simulink model "PLANET_v2"  (R2018b)
settings: Solver=FixedStepAuto  StartTime=0.0  StopTime=span-1  FixedStep=0.1  RelTol=1e-3
undefined symbols (not defined in the file): CHP_eta_el, CHP_eta_th, CHP_Pn, control, dh_demand, DH_elB_Cap, DH_elB_eff, DH_gas_B_Cap, DH_gas_B_eff, DH_HP_Cap, DH_HP_COP, DiscIntNeverNeededParam, dt, h_elD, lhd_demand, LHD_elB_Cap, LHD_elB_eff, LHD_gas_B_Cap, LHD_gas_B_eff, LHD_HP_Cap, LHD_HP_COP, Liion_cap, Liion_charge, Liion_dis, Liion_eff_ch, Liion_eff_dis, PCI, PtG_cap, PtG_eta_elcto, PtG_eta_meth, PtG_eta_th, PVPower, RES_curtailment_on_off, tt, WindPower
libraries: simulink x1
(part 2 of 5)

== system PLANET_v2/Control /Li-ion control/Max discharge rate MW ==
  Discharge capacity : Constant  Value=Max_discharge
  Max battery discharge : Outport
  wires:
  Discharge capacity/1 -> Max battery discharge/1

== system PLANET_v2/Control /Production to Demand/If Action Subsystem ==
  Power produced : Inport
  Power demand : Inport  Port=2
  Action Port : ActionPort  ActionType=then
  Constant : Constant  Value=0
  Sum : Sum  Inputs=|+-
  New demand : Outport
  Surplus : Outport  Port=2
  wires:
  Power produced/1 -> Sum/1
  Sum/1 -> Surplus/1
  Power demand/1 -> Sum/2
  Constant/1 -> New demand/1

== system PLANET_v2/Control /Production to Demand/If Action Subsystem1 ==
  Power produced : Inport
  Power demand : Inport  Port=2
  Action Port : ActionPort  ActionType=else
  Constant : Constant  Value=0
  Sum : Sum  Inputs=-+|
  Surplus : Outport
  New demand : Outport  Port=2
  wires:
  Sum/1 -> New demand/1
  Constant/1 -> Surplus/1
  Power demand/1 -> Sum/2
  Power produced/1 -> Sum/1

== system PLANET_v2/Control /Production to Demand1/If Action Subsystem ==
  Power produced : Inport
  Power demand : Inport  Port=2
  Action Port : ActionPort  ActionType=then
  Constant : Constant  Value=0
  Sum : Sum  Inputs=|+-
  New demand : Outport
  Surplus : Outport  Port=2
  wires:
  Power produced/1 -> Sum/1
  Sum/1 -> Surplus/1
  Power demand/1 -> Sum/2
  Constant/1 -> New demand/1

== system PLANET_v2/Control /Production to Demand1/If Action Subsystem1 ==
  Power produced : Inport
  Power demand : Inport  Port=2
  Action Port : ActionPort  ActionType=else
  Constant : Constant  Value=0
  Sum : Sum  Inputs=-+|
  Surplus : Outport
  New demand : Outport  Port=2
  wires:
  Sum/1 -> New demand/1
  Constant/1 -> Surplus/1
  Power demand/1 -> Sum/2
  Power produced/1 -> Sum/1

== system PLANET_v2/Control /Production to Demand2/If Action Subsystem ==
  Power produced : Inport
  Power demand : Inport  Port=2
  Action Port : ActionPort  ActionType=then
  Constant : Constant  Value=0
  Sum : Sum  Inputs=|+-
  New demand : Outport
  Surplus : Outport  Port=2
  wires:
  Power produced/1 -> Sum/1
  Sum/1 -> Surplus/1
  Power demand/1 -> Sum/2
  Constant/1 -> New demand/1

== system PLANET_v2/Control /Production to Demand2/If Action Subsystem1 ==
  Power produced : Inport
  Power demand : Inport  Port=2
  Action Port : ActionPort  ActionType=else
  Constant : Constant  Value=0
  Sum : Sum  Inputs=-+|
  Surplus : Outport
  New demand : Outport  Port=2
  wires:
  Sum/1 -> New demand/1
  Constant/1 -> Surplus/1
  Power demand/1 -> Sum/2
  Power produced/1 -> Sum/1

== system PLANET_v2/Control /Surplus dispacth/0: Li-ion P2G P2H1 ==
  Surplus MW : Inport
  " Li-ion charge MWh" : Inport  Port=2
  Th demand MW : Inport  Port=3
  Action Port : ActionPort  ActionType=then
  Li-ion control2 : Subsystem  mask{eff_charge=Liion_eff_ch, eff_discharge=Liion_eff_dis, SoC_MAX=100, SoC_MIN=0, Capacity=Liion_cap, Initial_SoC=50, Max_charge=Liion_charge, Max_discharge=Liion_dis}
      mask prompts: eff_charge "charging efficiency [%]"; eff_discharge "discharging efficiency [%]"; SoC_MAX "Maximum state of charge [%]"; SoC_MIN "Minimum state of charge [%]"; Capacity "Capacity [MWh]"; Initial_SoC "Initial State of charge [%]"; Max_charge "Max charge [MW]"; Max_discharge "Max discharge [MW]"
  P2G control : Subsystem  mask{PtG_capacity=PtG_cap, eff_electrolyser=PtG_eta_elcto, eff_methanizer=PtG_eta_meth, eff_thermal=PtG_eta_th, PCI=PCI}
      mask prompts: PtG_capacity "PtG capacity"; eff_electrolyser "Electrolyser efficiency"; eff_methanizer "Methanizer efficiency"; eff_thermal "Thermal efficiency"; PCI "PCI Mehtane MWh/kg"
  P2H : Subsystem  mask{HP_LHD_cap=LHD_HP_Cap, HP_LHD_COP=LHD_HP_COP, elB_LHD_cap=LHD_elB_Cap, elB_LHD_eff=LHD_elB_eff, HP_DH_cap=DH_HP_Cap, HP_DH_COP=DH_HP_COP, elB_DH_cap=DH_elB_Cap, elB_DH_eff=DH_elB_eff}
      mask prompts: HP_LHD_cap "LHD HP Capacity"; HP_LHD_COP "LHD HP COP"; elB_LHD_cap "LHD el boiler Capacity"; elB_LHD_eff "LHD el boiler efficiency"; HP_DH_cap "DH HP Capacity"; HP_DH_COP "DH HP COP"; elB_DH_cap "DH el boiler Capacity"; elB_DH_eff "DH el boiler efficiency"
  New surplus MW : Outport
  New th dem MW : Outport  Port=2
  Li-ion el input MW : Outport  Port=3
  P2G el input MW : Outport  Port=4
  P2H el input MW : Outport  Port=5
  wires:
  P2G control/1(New surplus MW) -> P2H/2(Surplus MW)
  Li-ion control2/1(New surplus MW) -> P2G control/1(Surplus MW)
  P2G control/2(P2G el input MW) -> P2G el input MW/1
  Li-ion control2/2(Battery el input MW) -> Li-ion el input MW/1
  " Li-ion charge MWh"/1 -> Li-ion control2/2(Initial charge MWh)
  P2H/3(New th dem) -> New th dem MW/1
  P2H/1(P2H el input) -> P2H el input MW/1
  P2H/2(New surplus MW) -> New surplus MW/1
  Th demand MW/1 -> P2H/1(Th demand)
  Surplus MW/1 -> Li-ion control2/1(Surplus MW)

== system PLANET_v2/Control /Surplus dispacth/1: Li-ion P2H P2G ==
  Surplus MW : Inport
  " Li-ion charge MWh" : Inport  Port=2
  Th demand MW : Inport  Port=3
  Action Port : ActionPort  ActionType=elseif
  Li-ion control2 : Subsystem  mask{eff_charge=Liion_eff_ch, eff_discharge=Liion_eff_dis, SoC_MAX=100, SoC_MIN=0, Capacity=Liion_cap, Initial_SoC=50, Max_charge=Liion_charge, Max_discharge=Liion_dis}
      mask prompts: eff_charge "charging efficiency [%]"; eff_discharge "discharging efficiency [%]"; SoC_MAX "Maximum state of charge [%]"; SoC_MIN "Minimum state of charge [%]"; Capacity "Capacity [MWh]"; Initial_SoC "Initial State of charge [%]"; Max_charge "Max charge [MW]"; Max_discharge "Max discharge [MW]"
  P2G control : Subsystem  mask{PtG_capacity=PtG_cap, eff_electrolyser=PtG_eta_elcto, eff_methanizer=PtG_eta_meth, eff_thermal=PtG_eta_th, PCI=PCI}
      mask prompts: PtG_capacity "PtG capacity"; eff_electrolyser "Electrolyser efficiency"; eff_methanizer "Methanizer efficiency"; eff_thermal "Thermal efficiency"; PCI "PCI Mehtane MWh/kg"
  P2H : Subsystem  mask{HP_LHD_cap=LHD_HP_Cap, HP_LHD_COP=LHD_HP_COP, elB_LHD_cap=LHD_elB_Cap, elB_LHD_eff=LHD_elB_eff, HP_DH_cap=DH_HP_Cap, HP_DH_COP=DH_HP_COP, elB_DH_cap=DH_elB_Cap, elB_DH_eff=DH_elB_eff}
      mask prompts: HP_LHD_cap "LHD HP Capacity"; HP_LHD_COP "LHD HP COP"; elB_LHD_cap "LHD el boiler Capacity"; elB_LHD_eff "LHD el boiler efficiency"; HP_DH_cap "DH HP Capacity"; HP_DH_COP "DH HP COP"; elB_DH_cap "DH el boiler Capacity"; elB_DH_eff "DH el boiler efficiency"
  New surplus MW : Outport
  New th dem MW : Outport  Port=2
  Li-ion el input MW : Outport  Port=3
  P2G el input MW : Outport  Port=4
  P2H el input MW : Outport  Port=5
  wires:
  P2G control/1(New surplus MW) -> New surplus MW/1
  P2H/2(New surplus MW) -> P2G control/1(Surplus MW)
  Li-ion control2/1(New surplus MW) -> P2H/2(Surplus MW)
  Surplus MW/1 -> Li-ion control2/1(Surplus MW)
  Th demand MW/1 -> P2H/1(Th demand)
  P2H/1(P2H el input) -> P2H el input MW/1
  P2H/3(New th dem) -> New th dem MW/1
  " Li-ion charge MWh"/1 -> Li-ion control2/2(Initial charge MWh)
  Li-ion control2/2(Battery el input MW) -> Li-ion el input MW/1
  P2G control/2(P2G el input MW) -> P2G el input MW/1

== system PLANET_v2/Control /Surplus dispacth/2: P2G Li-ion P2H ==
  Surplus MW : Inport
  " Li-ion charge MWh" : Inport  Port=2
  Th demand MW : Inport  Port=3
  Action Port : ActionPort  ActionType=elseif
  Li-ion control2 : Subsystem  mask{eff_charge=Liion_eff_ch, eff_discharge=Liion_eff_dis, SoC_MAX=100, SoC_MIN=0, Capacity=Liion_cap, Initial_SoC=50, Max_charge=Liion_charge, Max_discharge=Liion_dis}
      mask prompts: eff_charge "charging efficiency [%]"; eff_discharge "discharging efficiency [%]"; SoC_MAX "Maximum state of charge [%]"; SoC_MIN "Minimum state of charge [%]"; Capacity "Capacity [MWh]"; Initial_SoC "Initial State of charge [%]"; Max_charge "Max charge [MW]"; Max_discharge "Max discharge [MW]"
  P2G control : Subsystem  mask{PtG_capacity=PtG_cap, eff_electrolyser=PtG_eta_elcto, eff_methanizer=PtG_eta_meth, eff_thermal=PtG_eta_th, PCI=PCI}
      mask prompts: PtG_capacity "PtG capacity"; eff_electrolyser "Electrolyser efficiency"; eff_methanizer "Methanizer efficiency"; eff_thermal "Thermal efficiency"; PCI "PCI Mehtane MWh/kg"
  P2H : Subsystem  mask{HP_LHD_cap=LHD_HP_Cap, HP_LHD_COP=LHD_HP_COP, elB_LHD_cap=LHD_elB_Cap, elB_LHD_eff=LHD_elB_eff, HP_DH_cap=DH_HP_Cap, HP_DH_COP=DH_HP_COP, elB_DH_cap=DH_elB_Cap, elB_DH_eff=DH_elB_eff}
      mask prompts: HP_LHD_cap "LHD HP Capacity"; HP_LHD_COP "LHD HP COP"; elB_LHD_cap "LHD el boiler Capacity"; elB_LHD_eff "LHD el boiler efficiency"; HP_DH_cap "DH HP Capacity"; HP_DH_COP "DH HP COP"; elB_DH_cap "DH el boiler Capacity"; elB_DH_eff "DH el boiler efficiency"
  New surplus MW : Outport
  New th dem MW : Outport  Port=2
  Li-ion el input MW : Outport  Port=3
  P2G el input MW : Outport  Port=4
  P2H el input MW : Outport  Port=5
  wires:
  Li-ion control2/1(New surplus MW) -> P2H/2(Surplus MW)
  P2G control/1(New surplus MW) -> Li-ion control2/1(Surplus MW)
  Surplus MW/1 -> P2G control/1(Surplus MW)
  Th demand MW/1 -> P2H/1(Th demand)
  P2H/2(New surplus MW) -> New surplus MW/1
  P2H/1(P2H el input) -> P2H el input MW/1
  P2H/3(New th dem) -> New th dem MW/1
  " Li-ion charge MWh"/1 -> Li-ion control2/2(Initial charge MWh)
  Li-ion control2/2(Battery el input MW) -> Li-ion el input MW/1
  P2G control/2(P2G el input MW) -> P2G el input MW/1

== system PLANET_v2/Control /Surplus dispacth/3: P2G P2H Li-ion ==
  Surplus MW : Inport
  " Li-ion charge MWh" : Inport  Port=2
  Th demand MW : Inport  Port=3
  Action Port : ActionPort  ActionType=elseif
  Li-ion control2 : Subsystem  mask{eff_charge=Liion_eff_ch, eff_discharge=Liion_eff_dis, SoC_MAX=100, SoC_MIN=0, Capacity=Liion_cap, Initial_SoC=50, Max_charge=Liion_charge, Max_discharge=Liion_dis}
      mask prompts: eff_charge "charging efficiency [%]"; eff_discharge "discharging efficiency [%]"; SoC_MAX "Maximum state of charge [%]"; SoC_MIN "Minimum state of charge [%]"; Capacity "Capacity [MWh]"; Initial_SoC "Initial State of charge [%]"; Max_charge "Max charge [MW]"; Max_discharge "Max discharge [MW]"
  P2G control : Subsystem  mask{PtG_capacity=PtG_cap, eff_electrolyser=PtG_eta_elcto, eff_methanizer=PtG_eta_meth, eff_thermal=PtG_eta_th, PCI=PCI}
      mask prompts: PtG_capacity "PtG capacity"; eff_electrolyser "Electrolyser efficiency"; eff_methanizer "Methanizer efficiency"; eff_thermal "Thermal efficiency"; PCI "PCI Mehtane MWh/kg"
  P2H : Subsystem  mask{HP_LHD_cap=LHD_HP_Cap, HP_LHD_COP=LHD_HP_COP, elB_LHD_cap=LHD_elB_Cap, elB_LHD_eff=LHD_elB_eff, HP_DH_cap=DH_HP_Cap, HP_DH_COP=DH_HP_COP, elB_DH_cap=DH_elB_Cap, elB_DH_eff=DH_elB_eff}
      mask prompts: HP_LHD_cap "LHD HP Capacity"; HP_LHD_COP "LHD HP COP"; elB_LHD_cap "LHD el boiler Capacity"; elB_LHD_eff "LHD el boiler efficiency"; HP_DH_cap "DH HP Capacity"; HP_DH_COP "DH HP COP"; elB_DH_cap "DH el boiler Capacity"; elB_DH_eff "DH el boiler efficiency"
  New surplus MW : Outport
  New th dem MW : Outport  Port=2
  Li-ion el input MW : Outport  Port=3
  P2G el input MW : Outport  Port=4
  P2H el input MW : Outport  Port=5
  wires:
  Li-ion control2/1(New surplus MW) -> New surplus MW/1
  P2H/2(New surplus MW) -> Li-ion control2/1(Surplus MW)
  P2G control/1(New surplus MW) -> P2H/2(Surplus MW)
  Surplus MW/1 -> P2G control/1(Surplus MW)
  Th demand MW/1 -> P2H/1(Th demand)
  P2H/1(P2H el input) -> P2H el input MW/1
  P2H/3(New th dem) -> New th dem MW/1
  " Li-ion charge MWh"/1 -> Li-ion control2/2(Initial charge MWh)
  Li-ion control2/2(Battery el input MW) -> Li-ion el input MW/1
  P2G control/2(P2G el input MW) -> P2G el input MW/1

== system PLANET_v2/Control /Surplus dispacth/4: P2H Li-ion P2G ==
  Surplus MW : Inport
  " Li-ion charge MWh" : Inport  Port=2
  Th demand MW : Inport  Port=3
  Action Port : ActionPort  ActionType=elseif
  Li-ion control2 : Subsystem  mask{eff_charge=Liion_eff_ch, eff_discharge=Liion_eff_dis, SoC_MAX=100, SoC_MIN=0, Capacity=Liion_cap, Initial_SoC=50, Max_charge=Liion_charge, Max_discharge=Liion_dis}
      mask prompts: eff_charge "charging efficiency [%]"; eff_discharge "discharging efficiency [%]"; SoC_MAX "Maximum state of charge [%]"; SoC_MIN "Minimum state of charge [%]"; Capacity "Capacity [MWh]"; Initial_SoC "Initial State of charge [%]"; Max_charge "Max charge [MW]"; Max_discharge "Max discharge [MW]"
  P2G control : Subsystem  mask{PtG_capacity=PtG_cap, eff_electrolyser=PtG_eta_elcto, eff_methanizer=PtG_eta_meth, eff_thermal=PtG_eta_th, PCI=PCI}
      mask prompts: PtG_capacity "PtG capacity"; eff_electrolyser "Electrolyser efficiency"; eff_methanizer "Methanizer efficiency"; eff_thermal "Thermal efficiency"; PCI "PCI Mehtane MWh/kg"
  P2H : Subsystem  mask{HP_LHD_cap=LHD_HP_Cap, HP_LHD_COP=LHD_HP_COP, elB_LHD_cap=LHD_elB_Cap, elB_LHD_eff=LHD_elB_eff, HP_DH_cap=DH_HP_Cap, HP_DH_COP=DH_HP_COP, elB_DH_cap=DH_elB_Cap, elB_DH_eff=DH_elB_eff}
      mask prompts: HP_LHD_cap "LHD HP Capacity"; HP_LHD_COP "LHD HP COP"; elB_LHD_cap "LHD el boiler Capacity"; elB_LHD_eff "LHD el boiler efficiency"; HP_DH_cap "DH HP Capacity"; HP_DH_COP "DH HP COP"; elB_DH_cap "DH el boiler Capacity"; elB_DH_eff "DH el boiler efficiency"
  New surplus MW : Outport
  New th dem MW : Outport  Port=2
  Li-ion el input MW : Outport  Port=3
  P2G el input MW : Outport  Port=4
  P2H el input MW : Outport  Port=5
  wires:
  Surplus MW/1 -> P2H/2(Surplus MW)
  P2G control/1(New surplus MW) -> New surplus MW/1
  Li-ion control2/1(New surplus MW) -> P2G control/1(Surplus MW)
  P2H/2(New surplus MW) -> Li-ion control2/1(Surplus MW)
  Th demand MW/1 -> P2H/1(Th demand)
  P2H/1(P2H el input) -> P2H el input MW/1
  P2H/3(New th dem) -> New th dem MW/1
  " Li-ion charge MWh"/1 -> Li-ion control2/2(Initial charge MWh)
  Li-ion control2/2(Battery el input MW) -> Li-ion el input MW/1
  P2G control/2(P2G el input MW) -> P2G el input MW/1

== system PLANET_v2/Control /Surplus dispacth/5: P2H P2G Li-ion  ==
  Surplus MW : Inport
  " Li-ion charge MWh" : Inport  Port=2
  Th demand MW : Inport  Port=3
  Action Port : ActionPort  ActionType=elseif
  Li-ion control2 : Subsystem  mask{eff_charge=Liion_eff_ch, eff_discharge=Liion_eff_dis, SoC_MAX=100, SoC_MIN=0, Capacity=Liion_cap, Initial_SoC=50, Max_charge=Liion_charge, Max_discharge=Liion_dis}
      mask prompts: eff_charge "charging efficiency [%]"; eff_discharge "discharging efficiency [%]"; SoC_MAX "Maximum state of charge [%]"; SoC_MIN "Minimum state of charge [%]"; Capacity "Capacity [MWh]"; Initial_SoC "Initial State of charge [%]"; Max_charge "Max charge [MW]"; Max_discharge "Max discharge [MW]"
  P2G control : Subsystem  mask{PtG_capacity=PtG_cap, eff_electrolyser=PtG_eta_elcto, eff_methanizer=PtG_eta_meth, eff_thermal=PtG_eta_th, PCI=PCI}
      mask prompts: PtG_capacity "PtG capacity"; eff_electrolyser "Electrolyser efficiency"; eff_methanizer "Methanizer efficiency"; eff_thermal "Thermal efficiency"; PCI "PCI Mehtane MWh/kg"
  P2H : Subsystem  mask{HP_LHD_cap=LHD_HP_Cap, HP_LHD_COP=LHD_HP_COP, elB_LHD_cap=LHD_elB_Cap, elB_LHD_eff=LHD_elB_eff, HP_DH_cap=DH_HP_Cap, HP_DH_COP=DH_HP_COP, elB_DH_cap=DH_elB_Cap, elB_DH_eff=DH_elB_eff}
      mask prompts: HP_LHD_cap "LHD HP Capacity"; HP_LHD_COP "LHD HP COP"; elB_LHD_cap "LHD el boiler Capacity"; elB_LHD_eff "LHD el boiler efficiency"; HP_DH_cap "DH HP Capacity"; HP_DH_COP "DH HP COP"; elB_DH_cap "DH el boiler Capacity"; elB_DH_eff "DH el boiler efficiency"
  New surplus MW : Outport
  New th dem MW : Outport  Port=2
  Li-ion el input MW : Outport  Port=3
  P2G el input MW : Outport  Port=4
  P2H el input MW : Outport  Port=5
  wires:
  P2H/3(New th dem) -> New th dem MW/1
  Li-ion control2/1(New surplus MW) -> New surplus MW/1
  Surplus MW/1 -> P2H/2(Surplus MW)
  P2H/2(New surplus MW) -> P2G control/1(Surplus MW)
  P2G control/1(New surplus MW) -> Li-ion control2/1(Surplus MW)
  Th demand MW/1 -> P2H/1(Th demand)
  P2H/1(P2H el input) -> P2H el input MW/1
  " Li-ion charge MWh"/1 -> Li-ion control2/2(Initial charge MWh)
  Li-ion control2/2(Battery el input MW) -> Li-ion el input MW/1
  P2G control/2(P2G el input MW) -> P2G el input MW/1

== system PLANET_v2/Gas boiler (DH)/DH Gas Boiler block/Boiler ==
  Fuel mass : Inport
  Divide1 : Product  Inputs=***
  Efficiency : Constant  Value=eff/100
  PCI MWh/kg2 : Constant  Value=PCI
  Thermal power : Outport
  wires:
  Divide1/1 -> Thermal power/1
  Efficiency/1 -> Divide1/3
  Fuel mass/1 -> Divide1/1
  PCI MWh/kg2/1 -> Divide1/2

== system PLANET_v2/Gas boiler (LH)/LH Gas Boiler block/Boiler ==
  Fuel mass : Inport
  Divide1 : Product  Inputs=***
  Efficiency : Constant  Value=eff/100
  PCI MWh/kg2 : Constant  Value=PCI
  Thermal power : Outport
  wires:
  Divide1/1 -> Thermal power/1
  Efficiency/1 -> Divide1/3
  Fuel mass/1 -> Divide1/1
  PCI MWh/kg2/1 -> Divide1/2

== system PLANET_v2/Liion/Li-ion /State of charge calulation ==
  Charge : Inport
  Capacity : Constant  Value=Capacity
  Constant1 : Constant
  Divide : Product  Inputs=*/
  Gain : Gain  Gain=100
  Switch : Switch  Criteria=u2 > Threshold
  State of Charege : Outport
  wires:
  Charge/1 -> Divide/1
  Gain/1 -> State of Charege/1
  Divide/1 -> Gain/1
  Switch/1 -> Divide/2
  Capacity/1 -> Switch/2, Switch/1
  Constant1/1 -> Switch/3

== system PLANET_v2/Liion/Li-ion /Subsystem ==
  El input : Inport
  El output : Inport  Port=2
  Accumulation : DiscreteIntegrator  InitialConditionSource=external  ICPrevOutput=DiscIntNeverNeededParam  ICPrevScaledInput=DiscIntNeverNeededParam
  Initial Charge t0 : Subsystem
  Power to Energy : Subsystem
  Sum : Sum  Inputs=|++
  Sum1 : Sum  Inputs=+-|
  "Initial charge " : Outport
  New charge : Outport  Port=2
  wires:
  Sum/1 -> New charge/1
  Accumulation/1 -> "Initial charge "/1, Sum/2  "Charge inside the battery before the new input"
  Initial Charge t0/1(IC) -> Accumulation/2
  El input/1 -> Sum1/1
  El output/1 -> Sum1/2
  Power to Energy/1(Energy) -> Sum/1, Accumulation/1
  Sum1/1 -> Power to Energy/1(Power)

== system PLANET_v2/P2G/P2G/Max P2G electric input ==
  P2G capacity : Constant  Value=PtG_capacity
  Max P2G input : Outport
  wires:
  P2G capacity/1 -> Max P2G input/1

== system PLANET_v2/Subsystem/Environment/Analogic control1 ==
  Value : Inport
  Constant : Constant  Value=125.39682539683
  Constant1 : Constant  Value=0
  Gain : Gain  Gain=1/100
  Product : Product
  Switch : Switch  Criteria=u2 > Threshold
  Modifed value : Outport
  wires:
  Gain/1 -> Product/1
  Value/1 -> Switch/3, Product/2
  Switch/1 -> Modifed value/1
  Product/1 -> Switch/1
  Constant1/1 -> Switch/2
  Constant/1 -> Gain/1

== system PLANET_v2/Subsystem/Environment/Analogic control2 ==
  Value : Inport
  Constant : Constant  Value=100
  Constant1 : Constant  Value=0
  Gain : Gain  Gain=1/100
  Product : Product
  Switch : Switch  Criteria=u2 > Threshold
  Modifed value : Outport
  wires:
  Gain/1 -> Product/1
  Value/1 -> Switch/3, Product/2
  Switch/1 -> Modifed value/1
  Product/1 -> Switch/1
  Constant1/1 -> Switch/2
  Constant/1 -> Gain/1

== system PLANET_v2/Subsystem/Environment/Analogic control3 ==
  Value : Inport
  Constant : Constant  Value=100
  Constant1 : Constant  Value=0
  Gain : Gain  Gain=1/100
  Product : Product
  Switch : Switch  Criteria=u2 > Threshold
  Modifed value : Outport
  wires:
  Gain/1 -> Product/1
  Value/1 -> Switch/3, Product/2
  Switch/1 -> Modifed value/1
  Product/1 -> Switch/1
  Constant1/1 -> Switch/2
  Constant/1 -> Gain/1

== system PLANET_v2/Control /Surplus dispacth/0: Li-ion P2G P2H1/Li-ion control2 ==
  Surplus MW : Inport
  Initial charge MWh : Inport  Port=2
  " " : If  NumInputs=3  IfExpression=u1 == 0  ElseIfExpressions=(u1 <= u2) & (u1<=u3), u2<=u3
  Bypassed surp : Merge  Inputs=4
  Ch eff : Gain  Gain=100/eff_charge
  Charge to battery : Merge  Inputs=4
  Energy to Power : Subsystem
  Free Battery MWh : Subsystem
  If Action Subsystem : Subsystem  TreatAsAtomicUnit=on
  If Action Subsystem1 : Subsystem  TreatAsAtomicUnit=on
  If Action Subsystem2 : Subsystem  TreatAsAtomicUnit=on
  If Action Subsystem4 : Subsystem  TreatAsAtomicUnit=on
  MAX charge MW : Subsystem
  New surplus MW : Outport
  Battery el input MW : Outport  Port=2
  wires:
  Ch eff/1 -> " "/3, If Action Subsystem4/1(free battery)
  Energy to Power/1(Power) -> Ch eff/1
  Initial charge MWh/1 -> Free Battery MWh/1(In1)
  If Action Subsystem1/1(Bypassed surplus) -> Bypassed surp/2
  " "/2 -> If Action Subsystem1/Action
  If Action Subsystem/2(To battery) -> Charge to battery/1
  Free Battery MWh/1(Free space) -> Energy to Power/1(Energy)
  If Action Subsystem2/2(To battery) -> Charge to battery/3
  Surplus MW/1 -> If Action Subsystem1/1(Surplus), " "/1, If Action Subsystem2/2(Surplus), If Action Subsystem4/2(Surplus)
  " "/1 -> If Action Subsystem/Action
  If Action Subsystem4/2(To battery) -> Charge to battery/4
  " "/3 -> If Action Subsystem2/Action
  If Action Subsystem2/1(Bypassed surplus) -> Bypassed surp/3
  " "/4 -> If Action Subsystem4/Action
  Bypassed surp/1 -> New surplus MW/1  "Not accumulated energy surplus"
  If Action Subsystem1/2(To battery) -> Charge to battery/2
  Charge to battery/1 -> Battery el input MW/1  "Surplus energy send to the battery"
  MAX charge MW/1(Max battery charge) -> " "/2, If Action Subsystem2/1(Max charge)
  If Action Subsystem/1(Bypassed surplus) -> Bypassed surp/1
  If Action Subsystem4/1(Bypassed surplus) -> Bypassed surp/4

== system PLANET_v2/Control /Surplus dispacth/0: Li-ion P2G P2H1/P2G control ==
  Surplus MW : Inport
  If : If  NumInputs=2  IfExpression=u1 <= 0  ElseIfExpressions=u1 <= u2
  If Action Subsystem : Subsystem  TreatAsAtomicUnit=on
  If Action Subsystem1 : Subsystem  TreatAsAtomicUnit=on
  If Action Subsystem2 : Subsystem  TreatAsAtomicUnit=on
  Max P2G electric input : Subsystem
  Merge1 : Merge  Inputs=3
  Sum : Sum  Inputs=|+-
  New surplus MW : Outport
  P2G el input MW : Outport  Port=2
  wires:
  Max P2G electric input/1(Max PtG input) -> If/2
  If/1 -> If Action Subsystem2/Action
  If/3 -> If Action Subsystem/Action
  If Action Subsystem1/1(New surplus) -> Merge1/2
  Surplus MW/1 -> Sum/1, If Action Subsystem/1(Surplus), If/1
  If Action Subsystem/1(New surplus) -> Merge1/3
  If Action Subsystem2/1(New surplus) -> Merge1/1
  Merge1/1 -> Sum/2, New surplus MW/1
  If/2 -> If Action Subsystem1/Action
  Sum/1 -> P2G el input MW/1

== system PLANET_v2/Control /Surplus dispacth/0: Li-ion P2G P2H1/P2H ==
  Th demand : Inport
  Surplus MW : Inport  Port=2
  Bus Creator : BusCreator  Inputs=4
  Bus Creator1 : BusCreator  Inputs=2
  Bus Selector : BusSelector  OutputSignals=Lh dem,Dh dem
  Electric boiler DH : Subsystem  mask{th_eff=elB_DH_eff, Cap=elB_DH_cap}
      mask prompts: Cap "Capacity MW"
  Electric boiler LHD : Subsystem  mask{th_eff=elB_LHD_eff, Cap=elB_LHD_cap}
      mask prompts: Cap "Capacity MW"
  HEAT PUMP DH : Subsystem  mask{COP=HP_DH_COP, Cap=HP_DH_cap}
      mask prompts: Cap "Capacity MW"
  HEAT PUMP local : Subsystem  mask{COP=HP_LHD_COP, Cap=HP_LHD_cap}
      mask prompts: Cap "Capacity MW"
  P2H el input : Outport
  New surplus MW : Outport  Port=2
  New th dem : Outport  Port=3
  wires:
  Surplus MW/1 -> HEAT PUMP local/1(Surplus)
  Bus Selector/2 -> HEAT PUMP DH/2(th demand)  "<Dh dem>"
  HEAT PUMP local/2(New surplus) -> HEAT PUMP DH/1(Surplus)
  HEAT PUMP DH/2(New surplus) -> Electric boiler LHD/1(Surplus)
  HEAT PUMP local/3(New th_d) -> Electric boiler LHD/2(th demand)
  Electric boiler LHD/2(New surplus) -> Electric boiler DH/1(Surplus)
  HEAT PUMP DH/3(New th_d) -> Electric boiler DH/2(th demand)
  Electric boiler DH/2(New surplus) -> New surplus MW/1
  Electric boiler LHD/3(New th_d) -> Bus Creator1/1  "Lh dem"
  Electric boiler DH/3(New th_d) -> Bus Creator1/2  "Dh dem"
  HEAT PUMP local/1(el cons) -> Bus Creator/1  "HP (LH) el input"
  HEAT PUMP DH/1(el cons) -> Bus Creator/2  "HP (DH) el input"
  Electric boiler LHD/1(el cons) -> Bus Creator/3  "elB (LH) el input"
  Electric boiler DH/1(el cons) -> Bus Creator/4  "elB (DH) el input"
  Bus Creator/1 -> P2H el input/1
  Th demand/1 -> Bus Selector/1
  Bus Selector/1 -> HEAT PUMP local/2(th demand)  "<Lh dem>"
  Bus Creator1/1 -> New th dem/1  "Th dem"

== system PLANET_v2/Control /Surplus dispacth/1: Li-ion P2H P2G/Li-ion control2 ==
  Surplus MW : Inport
  Initial charge MWh : Inport  Port=2
  " " : If  NumInputs=3  IfExpression=u1 == 0  ElseIfExpressions=(u1 <= u2) & (u1<=u3), u2<=u3
  Bypassed surp : Merge  Inputs=4
  Ch eff : Gain  Gain=100/eff_charge
  Charge to battery : Merge  Inputs=4
  Energy to Power : Subsystem
  Free Battery MWh : Subsystem
  If Action Subsystem : Subsystem  TreatAsAtomicUnit=on
  If Action Subsystem1 : Subsystem  TreatAsAtomicUnit=on
  If Action Subsystem2 : Subsystem  TreatAsAtomicUnit=on
  If Action Subsystem4 : Subsystem  TreatAsAtomicUnit=on
  MAX charge MW : Subsystem
  New surplus MW : Outport
  Battery el input MW : Outport  Port=2
  wires:
  Ch eff/1 -> " "/3, If Action Subsystem4/1(free battery)
  Energy to Power/1(Power) -> Ch eff/1
  Initial charge MWh/1 -> Free Battery MWh/1(In1)
  If Action Subsystem1/1(Bypassed surplus) -> Bypassed surp/2
  " "/2 -> If Action Subsystem1/Action
  If Action Subsystem/2(To battery) -> Charge to battery/1
  Free Battery MWh/1(Free space) -> Energy to Power/1(Energy)
  If Action Subsystem2/2(To battery) -> Charge to battery/3
  Surplus MW/1 -> If Action Subsystem1/1(Surplus), " "/1, If Action Subsystem2/2(Surplus), If Action Subsystem4/2(Surplus)
  " "/1 -> If Action Subsystem/Action
  If Action Subsystem4/2(To battery) -> Charge to battery/4
  " "/3 -> If Action Subsystem2/Action
  If Action Subsystem2/1(Bypassed surplus) -> Bypassed surp/3
  " "/4 -> If Action Subsystem4/Action
  Bypassed surp/1 -> New surplus MW/1  "Not accumulated energy surplus"
  If Action Subsystem1/2(To battery) -> Charge to battery/2
  Charge to battery/1 -> Battery el input MW/1  "Surplus energy send to the battery"
  MAX charge MW/1(Max battery charge) -> " "/2, If Action Subsystem2/1(Max charge)
  If Action Subsystem/1(Bypassed surplus) -> Bypassed surp/1
  If Action Subsystem4/1(Bypassed surplus) -> Bypassed surp/4

== system PLANET_v2/Control /Surplus dispacth/1: Li-ion P2H P2G/P2G control ==
  Surplus MW : Inport
  If : If  NumInputs=2  IfExpression=u1 <= 0  ElseIfExpressions=u1 <= u2
  If Action Subsystem : Subsystem  TreatAsAtomicUnit=on
  If Action Subsystem1 : Subsystem  TreatAsAtomicUnit=on
  If Action Subsystem2 : Subsystem  TreatAsAtomicUnit=on
  Max P2G electric input : Subsystem
  Merge1 : Merge  Inputs=3
  Sum : Sum  Inputs=|+-
  New surplus MW : Outport
  P2G el input MW : Outport  Port=2
  wires:
  Max P2G electric input/1(Max PtG input) -> If/2
  If/1 -> If Action Subsystem2/Action
  If/3 -> If Action Subsystem/Action
  If Action Subsystem1/1(New surplus) -> Merge1/2
  Surplus MW/1 -> Sum/1, If Action Subsystem/1(Surplus), If/1
  If Action Subsystem/1(New surplus) -> Merge1/3
  If Action Subsystem2/1(New surplus) -> Merge1/1
  Merge1/1 -> Sum/2, New surplus MW/1
  If/2 -> If Action Subsystem1/Action
  Sum/1 -> P2G el input MW/1

== system PLANET_v2/Control /Surplus dispacth/1: Li-ion P2H P2G/P2H ==
  Th demand : Inport
  Surplus MW : Inport  Port=2
  Bus Creator : BusCreator  Inputs=4
  Bus Creator1 : BusCreator  Inputs=2
  Bus Selector : BusSelector  OutputSignals=Lh dem,Dh dem
  Electric boiler DH : Subsystem  mask{th_eff=elB_DH_eff, Cap=elB_DH_cap}
      mask prompts: Cap "Capacity MW"
  Electric boiler LHD : Subsystem  mask{th_eff=elB_LHD_eff, Cap=elB_LHD_cap}
      mask prompts: Cap "Capacity MW"
  HEAT PUMP DH : Subsystem  mask{COP=HP_DH_COP, Cap=HP_DH_cap}
      mask prompts: Cap "Capacity MW"
  HEAT PUMP local : Subsystem  mask{COP=HP_LHD_COP, Cap=HP_LHD_cap}
      mask prompts: Cap "Capacity MW"
  P2H el input : Outport
  New surplus MW : Outport  Port=2
  New th dem : Outport  Port=3
  wires:
  Bus Creator1/1 -> New th dem/1  "Th dem"
  Bus Selector/1 -> HEAT PUMP local/2(th demand)  "<Lh dem>"
  Th demand/1 -> Bus Selector/1
  Bus Creator/1 -> P2H el input/1
  Electric boiler DH/1(el cons) -> Bus Creator/4  "elB (DH) el input"
  Electric boiler LHD/1(el cons) -> Bus Creator/3  "elB (LH) el input"
  HEAT PUMP DH/1(el cons) -> Bus Creator/2  "HP (DH) el input"
  HEAT PUMP local/1(el cons) -> Bus Creator/1  "HP (LH) el input"
  Electric boiler DH/3(New th_d) -> Bus Creator1/2  "Dh dem"
  Electric boiler LHD/3(New th_d) -> Bus Creator1/1  "Lh dem"
  Electric boiler DH/2(New surplus) -> New surplus MW/1
  HEAT PUMP DH/3(New th_d) -> Electric boiler DH/2(th demand)
  Electric boiler LHD/2(New surplus) -> Electric boiler DH/1(Surplus)
  HEAT PUMP local/3(New th_d) -> Electric boiler LHD/2(th demand)
  HEAT PUMP DH/2(New surplus) -> Electric boiler LHD/1(Surplus)
  HEAT PUMP local/2(New surplus) -> HEAT PUMP DH/1(Surplus)
  Bus Selector/2 -> HEAT PUMP DH/2(th demand)  "<Dh dem>"
  Surplus MW/1 -> HEAT PUMP local/1(Surplus)

== system PLANET_v2/Control /Surplus dispacth/2: P2G Li-ion P2H/Li-ion control2 ==
  Surplus MW : Inport
  Initial charge MWh : Inport  Port=2
  " " : If  NumInputs=3  IfExpression=u1 == 0  ElseIfExpressions=(u1 <= u2) & (u1<=u3), u2<=u3
  Bypassed surp : Merge  Inputs=4
  Ch eff : Gain  Gain=100/eff_charge
  Charge to battery : Merge  Inputs=4
  Energy to Power : Subsystem
  Free Battery MWh : Subsystem
  If Action Subsystem : Subsystem  TreatAsAtomicUnit=on
  If Action Subsystem1 : Subsystem  TreatAsAtomicUnit=on
  If Action Subsystem2 : Subsystem  TreatAsAtomicUnit=on
  If Action Subsystem4 : Subsystem  TreatAsAtomicUnit=on
  MAX charge MW : Subsystem
  New surplus MW : Outport
  Battery el input MW : Outport  Port=2
  wires:
  Ch eff/1 -> " "/3, If Action Subsystem4/1(free battery)
  Energy to Power/1(Power) -> Ch eff/1
  Initial charge MWh/1 -> Free Battery MWh/1(In1)
  If Action Subsystem1/1(Bypassed surplus) -> Bypassed surp/2
  " "/2 -> If Action Subsystem1/Action
  If Action Subsystem/2(To battery) -> Charge to battery/1
  Free Battery MWh/1(Free space) -> Energy to Power/1(Energy)
  If Action Subsystem2/2(To battery) -> Charge to battery/3
  Surplus MW/1 -> If Action Subsystem1/1(Surplus), " "/1, If Action Subsystem2/2(Surplus), If Action Subsystem4/2(Surplus)
  " "/1 -> If Action Subsystem/Action
  If Action Subsystem4/2(To battery) -> Charge to battery/4
  " "/3 -> If Action Subsystem2/Action
  If Action Subsystem2/1(Bypassed surplus) -> Bypassed surp/3
  " "/4 -> If Action Subsystem4/Action
  Bypassed surp/1 -> New surplus MW/1  "Not accumulated energy surplus"
  If Action Subsystem1/2(To battery) -> Charge to battery/2
  Charge to battery/1 -> Battery el input MW/1  "Surplus energy send to the battery"
  MAX charge MW/1(Max battery charge) -> " "/2, If Action Subsystem2/1(Max charge)
  If Action Subsystem/1(Bypassed surplus) -> Bypassed surp/1
  If Action Subsystem4/1(Bypassed surplus) -> Bypassed surp/4

== system PLANET_v2/Control /Surplus dispacth/2: P2G Li-ion P2H/P2G control ==
  Surplus MW : Inport
  If : If  NumInputs=2  IfExpression=u1 <= 0  ElseIfExpressions=u1 <= u2
  If Action Subsystem : Subsystem  TreatAsAtomicUnit=on
  If Action Subsystem1 : Subsystem  TreatAsAtomicUnit=on
  If Action Subsystem2 : Subsystem  TreatAsAtomicUnit=on
  Max P2G electric input : Subsystem
  Merge1 : Merge  Inputs=3
  Sum : Sum  Inputs=|+-
  New surplus MW : Outport
  P2G el input MW : Outport  Port=2
  wires:
  Max P2G electric input/1(Max PtG input) -> If/2
  If/1 -> If Action Subsystem2/Action
  If/3 -> If Action Subsystem/Action
  If Action Subsystem1/1(New surplus) -> Merge1/2
  Surplus MW/1 -> Sum/1, If Action Subsystem/1(Surplus), If/1
  If Action Subsystem/1(New surplus) -> Merge1/3
  If Action Subsystem2/1(New surplus) -> Merge1/1
  Merge1/1 -> Sum/2, New surplus MW/1
  If/2 -> If Action Subsystem1/Action
  Sum/1 -> P2G el input MW/1

== system PLANET_v2/Control /Surplus dispacth/2: P2G Li-ion P2H/P2H ==
  Th demand : Inport
  Surplus MW : Inport  Port=2
  Bus Creator : BusCreator  Inputs=4
  Bus Creator1 : BusCreator  Inputs=2
  Bus Selector : BusSelector  OutputSignals=Lh dem,Dh dem
  Electric boiler DH : Subsystem  mask{th_eff=elB_DH_eff, Cap=elB_DH_cap}
      mask prompts: Cap "Capacity MW"
  Electric boiler LHD : Subsystem  mask{th_eff=elB_LHD_eff, Cap=elB_LHD_cap}
      mask prompts: Cap "Capacity MW"
  HEAT PUMP DH : Subsystem  mask{COP=HP_DH_COP, Cap=HP_DH_cap}
      mask prompts: Cap "Capacity MW"
  HEAT PUMP local : Subsystem  mask{COP=HP_LHD_COP, Cap=HP_LHD_cap}
      mask prompts: Cap "Capacity MW"
  P2H el input : Outport
  New surplus MW : Outport  Port=2
  New th dem : Outport  Port=3
  wires:
  Bus Creator1/1 -> New th dem/1  "Th dem"
  Bus Selector/1 -> HEAT PUMP local/2(th demand)  "<Lh dem>"
  Th demand/1 -> Bus Selector/1
  Bus Creator/1 -> P2H el input/1
  Electric boiler DH/1(el cons) -> Bus Creator/4  "elB (DH) el input"
  Electric boiler LHD/1(el cons) -> Bus Creator/3  "elB (LH) el input"
  HEAT PUMP DH/1(el cons) -> Bus Creator/2  "HP (DH) el input"
  HEAT PUMP local/1(el cons) -> Bus Creator/1  "HP (LH) el input"
  Electric boiler DH/3(New th_d) -> Bus Creator1/2  "Dh dem"
  Electric boiler LHD/3(New th_d) -> Bus Creator1/1  "Lh dem"
  Electric boiler DH/2(New surplus) -> New surplus MW/1
  HEAT PUMP DH/3(New th_d) -> Electric boiler DH/2(th demand)
  Electric boiler LHD/2(New surplus) -> Electric boiler DH/1(Surplus)
  HEAT PUMP local/3(New th_d) -> Electric boiler LHD/2(th demand)
  HEAT PUMP DH/2(New surplus) -> Electric boiler LHD/1(Surplus)
  HEAT PUMP local/2(New surplus) -> HEAT PUMP DH/1(Surplus)
  Bus Selector/2 -> HEAT PUMP DH/2(th demand)  "<Dh dem>"
  Surplus MW/1 -> HEAT PUMP local/1(Surplus)

== system PLANET_v2/Control /Surplus dispacth/3: P2G P2H Li-ion/Li-ion control2 ==
  Surplus MW : Inport
  Initial charge MWh : Inport  Port=2
  " " : If  NumInputs=3  IfExpression=u1 == 0  ElseIfExpressions=(u1 <= u2) & (u1<=u3), u2<=u3
  Bypassed surp : Merge  Inputs=4
  Ch eff : Gain  Gain=100/eff_charge
  Charge to battery : Merge  Inputs=4
  Energy to Power : Subsystem
  Free Battery MWh : Subsystem
  If Action Subsystem : Subsystem  TreatAsAtomicUnit=on
  If Action Subsystem1 : Subsystem  TreatAsAtomicUnit=on
  If Action Subsystem2 : Subsystem  TreatAsAtomicUnit=on
  If Action Subsystem4 : Subsystem  TreatAsAtomicUnit=on
  MAX charge MW : Subsystem
  New surplus MW : Outport
  Battery el input MW : Outport  Port=2
  wires:
  Ch eff/1 -> " "/3, If Action Subsystem4/1(free battery)
  Energy to Power/1(Power) -> Ch eff/1
  Initial charge MWh/1 -> Free Battery MWh/1(In1)
  If Action Subsystem1/1(Bypassed surplus) -> Bypassed surp/2
  " "/2 -> If Action Subsystem1/Action
  If Action Subsystem/2(To battery) -> Charge to battery/1
  Free Battery MWh/1(Free space) -> Energy to Power/1(Energy)
  If Action Subsystem2/2(To battery) -> Charge to battery/3
  Surplus MW/1 -> If Action Subsystem1/1(Surplus), " "/1, If Action Subsystem2/2(Surplus), If Action Subsystem4/2(Surplus)
  " "/1 -> If Action Subsystem/Action
  If Action Subsystem4/2(To battery) -> Charge to battery/4
  " "/3 -> If Action Subsystem2/Action
  If Action Subsystem2/1(Bypassed surplus) -> Bypassed surp/3
  " "/4 -> If Action Subsystem4/Action
  Bypassed surp/1 -> New surplus MW/1  "Not accumulated energy surplus"
  If Action Subsystem1/2(To battery) -> Charge to battery/2
  Charge to battery/1 -> Battery el input MW/1  "Surplus energy send to the battery"
  MAX charge MW/1(Max battery charge) -> " "/2, If Action Subsystem2/1(Max charge)
  If Action Subsystem/1(Bypassed surplus) -> Bypassed surp/1
  If Action Subsystem4/1(Bypassed surplus) -> Bypassed surp/4

== system PLANET_v2/Control /Surplus dispacth/3: P2G P2H Li-ion/P2G control ==
  Surplus MW : Inport
  If : If  NumInputs=2  IfExpression=u1 <= 0  ElseIfExpressions=u1 <= u2
  If Action Subsystem : Subsystem  TreatAsAtomicUnit=on
  If Action Subsystem1 : Subsystem  TreatAsAtomicUnit=on
  If Action Subsystem2 : Subsystem  TreatAsAtomicUnit=on
  Max P2G electric input : Subsystem
  Merge1 : Merge  Inputs=3
  Sum : Sum  Inputs=|+-
  New surplus MW : Outport
  P2G el input MW : Outport  Port=2
  wires:
  Max P2G electric input/1(Max PtG input) -> If/2
  If/1 -> If Action Subsystem2/Action
  If/3 -> If Action Subsystem/Action
  If Action Subsystem1/1(New surplus) -> Merge1/2
  Surplus MW/1 -> Sum/1, If Action Subsystem/1(Surplus), If/1
  If Action Subsystem/1(New surplus) -> Merge1/3
  If Action Subsystem2/1(New surplus) -> Merge1/1
  Merge1/1 -> Sum/2, New surplus MW/1
  If/2 -> If Action Subsystem1/Action
  Sum/1 -> P2G el input MW/1

== system PLANET_v2/Control /Surplus dispacth/3: P2G P2H Li-ion/P2H ==
  Th demand : Inport
  Surplus MW : Inport  Port=2
  Bus Creator : BusCreator  Inputs=4
  Bus Creator1 : BusCreator  Inputs=2
  Bus Selector : BusSelector  OutputSignals=Lh dem,Dh dem
  Electric boiler DH : Subsystem  mask{th_eff=elB_DH_eff, Cap=elB_DH_cap}
      mask prompts: Cap "Capacity MW"
  Electric boiler LHD : Subsystem  mask{th_eff=elB_LHD_eff, Cap=elB_LHD_cap}
      mask prompts: Cap "Capacity MW"
  HEAT PUMP DH : Subsystem  mask{COP=HP_DH_COP, Cap=HP_DH_cap}
      mask prompts: Cap "Capacity MW"
  HEAT PUMP local : Subsystem  mask{COP=HP_LHD_COP, Cap=HP_LHD_cap}
      mask prompts: Cap "Capacity MW"
  P2H el input : Outport
  New surplus MW : Outport  Port=2
  New th dem : Outport  Port=3
  wires:
  Bus Creator1/1 -> New th dem/1  "Th dem"
  Bus Selector/1 -> HEAT PUMP local/2(th demand)  "<Lh dem>"
  Th demand/1 -> Bus Selector/1
  Bus Creator/1 -> P2H el input/1
  Electric boiler DH/1(el cons) -> Bus Creator/4  "elB (DH) el input"
  Electric boiler LHD/1(el cons) -> Bus Creator/3  "elB (LH) el input"
  HEAT PUMP DH/1(el cons) -> Bus Creator/2  "HP (DH) el input"
  HEAT PUMP local/1(el cons) -> Bus Creator/1  "HP (LH) el input"
  Electric boiler DH/3(New th_d) -> Bus Creator1/2  "Dh dem"
  Electric boiler LHD/3(New th_d) -> Bus Creator1/1  "Lh dem"
  Electric boiler DH/2(New surplus) -> New surplus MW/1
  HEAT PUMP DH/3(New th_d) -> Electric boiler DH/2(th demand)
  Electric boiler LHD/2(New surplus) -> Electric boiler DH/1(Surplus)
  HEAT PUMP local/3(New th_d) -> Electric boiler LHD/2(th demand)
  HEAT PUMP DH/2(New surplus) -> Electric boiler LHD/1(Surplus)
  HEAT PUMP local/2(New surplus) -> HEAT PUMP DH/1(Surplus)
  Bus Selector/2 -> HEAT PUMP DH/2(th demand)  "<Dh dem>"
  Surplus MW/1 -> HEAT PUMP local/1(Surplus)

== system PLANET_v2/Control /Surplus dispacth/4: P2H Li-ion P2G/Li-ion control2 ==
  Surplus MW : Inport
  Initial charge MWh : Inport  Port=2
  " " : If  NumInputs=3  IfExpression=u1 == 0  ElseIfExpressions=(u1 <= u2) & (u1<=u3), u2<=u3
  Bypassed surp : Merge  Inputs=4
  Ch eff : Gain  Gain=100/eff_charge
  Charge to battery : Merge  Inputs=4
  Energy to Power : Subsystem
  Free Battery MWh : Subsystem
  If Action Subsystem : Subsystem  TreatAsAtomicUnit=on
  If Action Subsystem1 : Subsystem  TreatAsAtomicUnit=on
  If Action Subsystem2 : Subsystem  TreatAsAtomicUnit=on
  If Action Subsystem4 : Subsystem  TreatAsAtomicUnit=on
  MAX charge MW : Subsystem
  New surplus MW : Outport
  Battery el input MW : Outport  Port=2
  wires:
  Ch eff/1 -> " "/3, If Action Subsystem4/1(free battery)
  Energy to Power/1(Power) -> Ch eff/1
  Initial charge MWh/1 -> Free Battery MWh/1(In1)
  If Action Subsystem1/1(Bypassed surplus) -> Bypassed surp/2
  " "/2 -> If Action Subsystem1/Action
  If Action Subsystem/2(To battery) -> Charge to battery/1
  Free Battery MWh/1(Free space) -> Energy to Power/1(Energy)
  If Action Subsystem2/2(To battery) -> Charge to battery/3
  Surplus MW/1 -> If Action Subsystem1/1(Surplus), " "/1, If Action Subsystem2/2(Surplus), If Action Subsystem4/2(Surplus)
  " "/1 -> If Action Subsystem/Action
  If Action Subsystem4/2(To battery) -> Charge to battery/4
  " "/3 -> If Action Subsystem2/Action
  If Action Subsystem2/1(Bypassed surplus) -> Bypassed surp/3
  " "/4 -> If Action Subsystem4/Action
  Bypassed surp/1 -> New surplus MW/1  "Not accumulated energy surplus"
  If Action Subsystem1/2(To battery) -> Charge to battery/2
  Charge to battery/1 -> Battery el input MW/1  "Surplus energy send to the battery"
  MAX charge MW/1(Max battery charge) -> " "/2, If Action Subsystem2/1(Max charge)
  If Action Subsystem/1(Bypassed surplus) -> Bypassed surp/1
  If Action Subsystem4/1(Bypassed surplus) -> Bypassed surp/4

== system PLANET_v2/Control /Surplus dispacth/4: P2H Li-ion P2G/P2G control ==
  Surplus MW : Inport
  If : If  NumInputs=2  IfExpression=u1 <= 0  ElseIfExpressions=u1 <= u2
  If Action Subsystem : Subsystem  TreatAsAtomicUnit=on
  If Action Subsystem1 : Subsystem  TreatAsAtomicUnit=on
  If Action Subsystem2 : Subsystem  TreatAsAtomicUnit=on
  Max P2G electric input : Subsystem
  Merge1 : Merge  Inputs=3
  Sum : Sum  Inputs=|+-
  New surplus MW : Outport
  P2G el input MW : Outport  Port=2
  wires:
  Max P2G electric input/1(Max PtG input) -> If/2
  If/1 -> If Action Subsystem2/Action
  If/3 -> If Action Subsystem/Action
  If Action Subsystem1/1(New surplus) -> Merge1/2
  Surplus MW/1 -> Sum/1, If Action Subsystem/1(Surplus), If/1
  If Action Subsystem/1(New surplus) -> Merge1/3
  If Action Subsystem2/1(New surplus) -> Merge1/1
  Merge1/1 -> Sum/2, New surplus MW/1
  If/2 -> If Action Subsystem1/Action
  Sum/1 -> P2G el input MW/1

== system PLANET_v2/Control /Surplus dispacth/4: P2H Li-ion P2G/P2H ==
  Th demand : Inport
  Surplus MW : Inport  Port=2
  Bus Creator : BusCreator  Inputs=4
  Bus Creator1 : BusCreator  Inputs=2
  Bus Selector : BusSelector  OutputSignals=Lh dem,Dh dem
  Electric boiler DH : Subsystem  mask{th_eff=elB_DH_eff, Cap=elB_DH_cap}
      mask prompts: Cap "Capacity MW"
  Electric boiler LHD : Subsystem  mask{th_eff=elB_LHD_eff, Cap=elB_LHD_cap}
      mask prompts: Cap "Capacity MW"
  HEAT PUMP DH : Subsystem  mask{COP=HP_DH_COP, Cap=HP_DH_cap}
      mask prompts: Cap "Capacity MW"
  HEAT PUMP local : Subsystem  mask{COP=HP_LHD_COP, Cap=HP_LHD_cap}
      mask prompts: Cap "Capacity MW"
  P2H el input : Outport
  New surplus MW : Outport  Port=2
  New th dem : Outport  Port=3
  wires:
  Bus Creator1/1 -> New th dem/1  "Th dem"
  Bus Selector/1 -> HEAT PUMP local/2(th demand)  "<Lh dem>"
  Th demand/1 -> Bus Selector/1
  Bus Creator/1 -> P2H el input/1
  Electric boiler DH/1(el cons) -> Bus Creator/4  "elB (DH) el input"
  Electric boiler LHD/1(el cons) -> Bus Creator/3  "elB (LH) el input"
  HEAT PUMP DH/1(el cons) -> Bus Creator/2  "HP (DH) el input"
  HEAT PUMP local/1(el cons) -> Bus Creator/1  "HP (LH) el input"
  Electric boiler DH/3(New th_d) -> Bus Creator1/2  "Dh dem"
  Electric boiler LHD/3(New th_d) -> Bus Creator1/1  "Lh dem"
  Electric boiler DH/2(New surplus) -> New surplus MW/1
  HEAT PUMP DH/3(New th_d) -> Electric boiler DH/2(th demand)
  Electric boiler LHD/2(New surplus) -> Electric boiler DH/1(Surplus)
  HEAT PUMP local/3(New th_d) -> Electric boiler LHD/2(th demand)
  HEAT PUMP DH/2(New surplus) -> Electric boiler LHD/1(Surplus)
  HEAT PUMP local/2(New surplus) -> HEAT PUMP DH/1(Surplus)
  Bus Selector/2 -> HEAT PUMP DH/2(th demand)  "<Dh dem>"
  Surplus MW/1 -> HEAT PUMP local/1(Surplus)

== system PLANET_v2/Control /Surplus dispacth/5: P2H P2G Li-ion /Li-ion control2 ==
  Surplus MW : Inport
  Initial charge MWh : Inport  Port=2
  " " : If  NumInputs=3  IfExpression=u1 == 0  ElseIfExpressions=(u1 <= u2) & (u1<=u3), u2<=u3
  Bypassed surp : Merge  Inputs=4
  Ch eff : Gain  Gain=100/eff_charge
  Charge to battery : Merge  Inputs=4
  Energy to Power : Subsystem
  Free Battery MWh : Subsystem
  If Action Subsystem : Subsystem  TreatAsAtomicUnit=on
  If Action Subsystem1 : Subsystem  TreatAsAtomicUnit=on
  If Action Subsystem2 : Subsystem  TreatAsAtomicUnit=on
  If Action Subsystem4 : Subsystem  TreatAsAtomicUnit=on
  MAX charge MW : Subsystem
  New surplus MW : Outport
  Battery el input MW : Outport  Port=2
  wires:
  Ch eff/1 -> " "/3, If Action Subsystem4/1(free battery)
  Energy to Power/1(Power) -> Ch eff/1
  Initial charge MWh/1 -> Free Battery MWh/1(In1)
  If Action Subsystem1/1(Bypassed surplus) -> Bypassed surp/2
  " "/2 -> If Action Subsystem1/Action
  If Action Subsystem/2(To battery) -> Charge to battery/1
  Free Battery MWh/1(Free space) -> Energy to Power/1(Energy)
  If Action Subsystem2/2(To battery) -> Charge to battery/3
  Surplus MW/1 -> If Action Subsystem1/1(Surplus), " "/1, If Action Subsystem2/2(Surplus), If Action Subsystem4/2(Surplus)
  " "/1 -> If Action Subsystem/Action
  If Action Subsystem4/2(To battery) -> Charge to battery/4
  " "/3 -> If Action Subsystem2/Action
  If Action Subsystem2/1(Bypassed surplus) -> Bypassed surp/3
  " "/4 -> If Action Subsystem4/Action
  Bypassed surp/1 -> New surplus MW/1  "Not accumulated energy surplus"
  If Action Subsystem1/2(To battery) -> Charge to battery/2
  Charge to battery/1 -> Battery el input MW/1  "Surplus energy send to the battery"
  MAX charge MW/1(Max battery charge) -> " "/2, If Action Subsystem2/1(Max charge)
  If Action Subsystem/1(Bypassed surplus) -> Bypassed surp/1
  If Action Subsystem4/1(Bypassed surplus) -> Bypassed surp/4

== system PLANET_v2/Control /Surplus dispacth/5: P2H P2G Li-ion /P2G control ==
  Surplus MW : Inport
  If : If  NumInputs=2  IfExpression=u1 <= 0  ElseIfExpressions=u1 <= u2
  If Action Subsystem : Subsystem  TreatAsAtomicUnit=on
  If Action Subsystem1 : Subsystem  TreatAsAtomicUnit=on
  If Action Subsystem2 : Subsystem  TreatAsAtomicUnit=on
  Max P2G electric input : Subsystem
  Merge1 : Merge  Inputs=3
  Sum : Sum  Inputs=|+-
  New surplus MW : Outport
  P2G el input MW : Outport  Port=2
  wires:
  Max P2G electric input/1(Max PtG input) -> If/2
  If/1 -> If Action Subsystem2/Action
  If/3 -> If Action Subsystem/Action
  If Action Subsystem1/1(New surplus) -> Merge1/2
  Surplus MW/1 -> Sum/1, If Action Subsystem/1(Surplus), If/1
  If Action Subsystem/1(New surplus) -> Merge1/3
  If Action Subsystem2/1(New surplus) -> Merge1/1
  Merge1/1 -> Sum/2, New surplus MW/1
  If/2 -> If Action Subsystem1/Action
  Sum/1 -> P2G el input MW/1

== system PLANET_v2/Control /Surplus dispacth/5: P2H P2G Li-ion /P2H ==
  Th demand : Inport
  Surplus MW : Inport  Port=2
  Bus Creator : BusCreator  Inputs=4
  Bus Creator1 : BusCreator  Inputs=2
  Bus Selector : BusSelector  OutputSignals=Lh dem,Dh dem
  Electric boiler DH : Subsystem  mask{th_eff=elB_DH_eff, Cap=elB_DH_cap}
      mask prompts: Cap "Capacity MW"
  Electric boiler LHD : Subsystem  mask{th_eff=elB_LHD_eff, Cap=elB_LHD_cap}
      mask prompts: Cap "Capacity MW"
  HEAT PUMP DH : Subsystem  mask{COP=HP_DH_COP, Cap=HP_DH_cap}
      mask prompts: Cap "Capacity MW"
  HEAT PUMP local : Subsystem  mask{COP=HP_LHD_COP, Cap=HP_LHD_cap}
      mask prompts: Cap "Capacity MW"
  P2H el input : Outport
  New surplus MW : Outport  Port=2
  New th dem : Outport  Port=3
  wires:
  Bus Creator1/1 -> New th dem/1  "Th dem"
  Bus Selector/1 -> HEAT PUMP local/2(th demand)  "<Lh dem>"
  Th demand/1 -> Bus Selector/1
  Bus Creator/1 -> P2H el input/1
  Electric boiler DH/1(el cons) -> Bus Creator/4  "elB (DH) el input"
  Electric boiler LHD/1(el cons) -> Bus Creator/3  "elB (LH) el input"
  HEAT PUMP DH/1(el cons) -> Bus Creator/2  "HP (DH) el input"
  HEAT PUMP local/1(el cons) -> Bus Creator/1  "HP (LH) el input"
  Electric boiler DH/3(New th_d) -> Bus Creator1/2  "Dh dem"
  Electric boiler LHD/3(New th_d) -> Bus Creator1/1  "Lh dem"
  Electric boiler DH/2(New surplus) -> New surplus MW/1
  HEAT PUMP DH/3(New th_d) -> Electric boiler DH/2(th demand)
  Electric boiler LHD/2(New surplus) -> Electric boiler DH/1(Surplus)
  HEAT PUMP local/3(New th_d) -> Electric boiler LHD/2(th demand)
  HEAT PUMP DH/2(New surplus) -> Electric boiler LHD/1(Surplus)
  HEAT PUMP local/2(New surplus) -> HEAT PUMP DH/1(Surplus)
  Bus Selector/2 -> HEAT PUMP DH/2(th demand)  "<Dh dem>"
  Surplus MW/1 -> HEAT PUMP local/1(Surplus)

== system PLANET_v2/Liion/Li-ion /Subsystem/Initial Charge t0 ==
  Capacity [MWh] : Constant  Value=Capacity
  Initial SoC [%] : Constant  Value=Initial_SoC/100
  Product2 : Product
  IC : Outport
  wires:
  Capacity [MWh]/1 -> Product2/1
  Initial SoC [%]/1 -> Product2/2
  Product2/1 -> IC/1

== system PLANET_v2/Liion/Li-ion /Subsystem/Power to Energy ==
  Power : Inport
  Power to Energy : Gain  Gain=dt
  Energy : Outport
  wires:
  Power/1 -> Power to Energy/1
  Power to Energy/1 -> Energy/1

== system PLANET_v2/Control /Surplus dispacth/0: Li-ion P2G P2H1/Li-ion control2/Energy to Power ==
  Energy : Inport
  Energy to Power : Gain  Gain=1/dt
  Power : Outport
  wires:
  Energy to Power/1 -> Power/1
  Energy/1 -> Energy to Power/1

== system PLANET_v2/Control /Surplus dispacth/0: Li-ion P2G P2H1/Li-ion control2/Free Battery MWh ==
  In1 : Inport
  Capacity [MWh] : Constant  Value=Capacity
  Product : Product
  Steate of Charge MAX [%] : Constant  Value=SoC_MAX/100
  Sum : Sum  Inputs=+|-
  Free space : Outport
  wires:
  Product/1 -> Sum/1
  Steate of Charge MAX [%]/1 -> Product/1
  Capacity [MWh]/1 -> Product/2
  Sum/1 -> Free space/1
  In1/1 -> Sum/2

== system PLANET_v2/Control /Surplus dispacth/0: Li-ion P2G P2H1/Li-ion control2/If Action Subsystem ==
  Action Port : ActionPort  ActionType=then
  Constant : Constant  Value=0
  Bypassed surplus : Outport
  To battery : Outport  Port=2
  wires:
  Constant/1 -> To battery/1, Bypassed surplus/1
